simulink model "Paper_2_Model_2_3_lines_of_delays_with_PDF_Gaussian"  (R2020b)
settings: Solver=VariableStepAuto  StartTime=0.0  StopTime=10.0  RelTol=1e-3
libraries: simulink x1
settings Model: Creator=Isabel  LastModifiedBy=Isabel

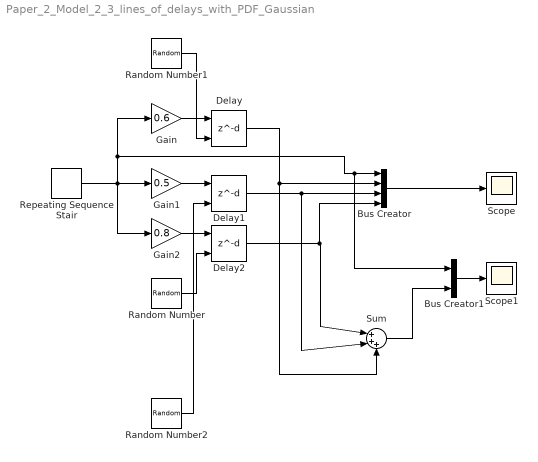
== system Paper_2_Model_2_3_lines_of_delays_with_PDF_Gaussian ==
  Bus Creator : BusCreator  Inputs=4
  Bus Creator1 : BusCreator  Inputs=2
  Delay : Delay  DelayLengthSource=Input port  InitialCondition=0  UseCircularBuffer=on  SampleTime=0.05
      settings: InputPortMap=u0,p1
  Delay1 : Delay  DelayLengthSource=Input port  DelayLength=10  InitialCondition=0  SampleTime=0.05
      settings: InputPortMap=u0,p1
  Delay2 : Delay  DelayLengthSource=Input port  DelayLength=4  InitialCondition=0  SampleTime=0.05
      settings: InputPortMap=u0,p1
  Gain : Gain  Gain=0.6
  Gain1 : Gain  Gain=0.5
  Gain2 : Gain  Gain=0.8
  Random Number : RandomNumber  Mean=2  Variance=4  SampleTime=3
  Random Number1 : RandomNumber  Mean=10  Variance=4  SampleTime=3
  Random Number2 : RandomNumber  Mean=15  Variance=5  Seed=1  SampleTime=3
  Repeating Sequence Stair : simulink/Sources/Repeating Sequence Stair  OutValues=[0 0 0 1 0 0 0 1 0 0 0 1 0 0 0 1 0 0 0].'  tsamp=0.5  OutMin=[]  OutMax=[]  OutDataTypeStr=double  OutputDataTypeScalingMode=double  OutDataType=fixdt(0,8)  ConRadixGroup=Best Precision: Vector-wise  OutScaling=2^-12
  Scope : Scope
  Scope1 : Scope
  Sum : Sum  Inputs=|+++
  wires:
  Gain/1 -> Delay/1
  Gain2/1 -> Delay2/1
  Delay2/1 -> Bus Creator/4, Sum/1
  Bus Creator/1 -> Scope/1
  Gain1/1 -> Delay1/1
  Random Number/1 -> Delay2/2
  Delay1/1 -> Bus Creator/3, Sum/2
  Delay/1 -> Bus Creator/2, Sum/3
  Random Number2/1 -> Delay1/2
  Sum/1 -> Bus Creator1/2
  Bus Creator1/1 -> Scope1/1
  Repeating Sequence Stair/1 -> Bus Creator1/1, Bus Creator/1, Gain/1, Gain2/1, Gain1/1
  Random Number1/1 -> Delay/2
